simulink model "Motion_Planning"  (R2023b)
settings: Solver=VariableStepAuto  StartTime=0.0  StopTime=10.0  RelTol=1e-3
undefined symbols (not defined in the file or in its folder): Spline_Max_Centripital_Acceleration, Spline_Max_Linear_Acceleration, Spline_Max_Num_RefPoses, Spline_Max_Speed, Spline_Num_Samples
libraries: simulink x10
settings Model: Creator=FIRSTMentor  LastModifiedBy=FIRSTMentor

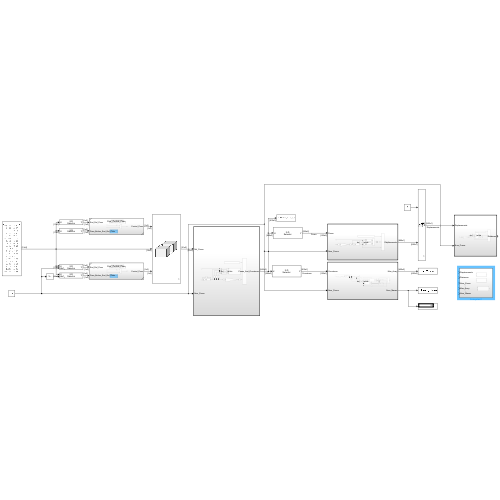
[thumbnail: Simulink's stored preview of the top-level diagram]
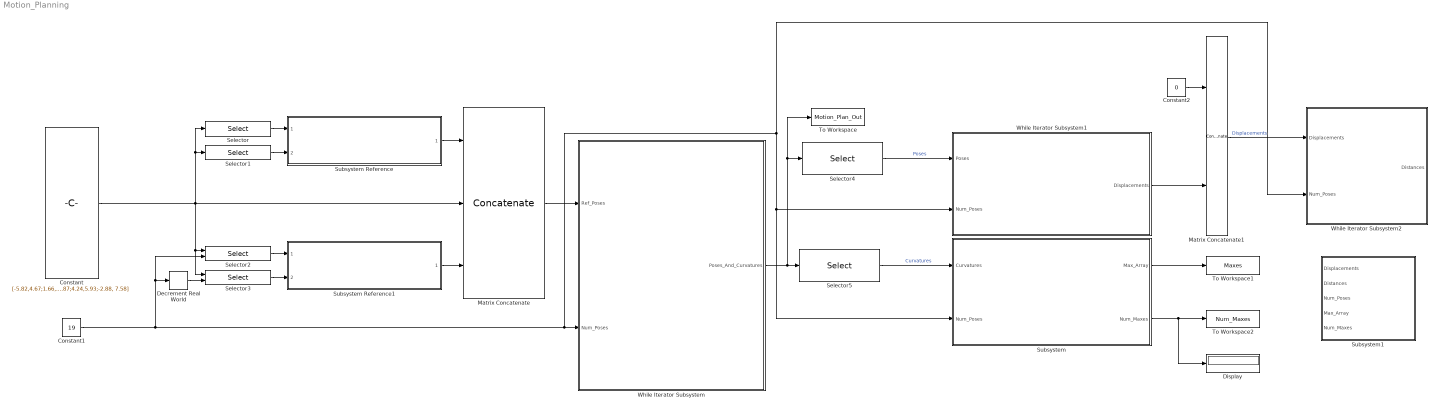
== system Motion_Planning ==
  Constant : Constant  Value=[-5.82,4.67;1.66,4.85;5,3.79;4.44,2.57;-5.94,2.47;-6.48,1.59;-5.46,0.81;4.2,0.75;-5.46,-0.25;3.9,-1.37;2.52,-2.81;5.36,-3.05;2.44,-4.71;-6.24,-4.09;-7.4,-2.43;-7.94,4.19;-7.6,5.87;4.24,5.93;-2.88, 7.58]  VectorParams1D=off
  Constant1 : Constant  Value=19
  Constant2 : Constant  Value=0
  Decrement Real World : simulink/Additional Math & Discrete/Additional Math: Increment - Decrement/Decrement Real World
  Display : Display
  Matrix Concatenate : Concatenate  NumInputs=3  Mode=Multidimensional array
  Matrix Concatenate1 : Concatenate  Mode=Multidimensional array
  Selector : Selector  NumberOfDimensions=2  InputPortWidth=3  IndexOptions=Index vector (dialog),Select all  Indices=1,1  OutputSizes=1,1
  Selector1 : Selector  NumberOfDimensions=2  InputPortWidth=3  IndexOptions=Index vector (dialog),Select all  Indices=2,1  OutputSizes=1,1
  Selector2 : Selector  NumberOfDimensions=2  InputPortWidth=3  IndexOptions=Index vector (port),Select all  Indices=[1 3],1  OutputSizes=1,1
  Selector3 : Selector  NumberOfDimensions=2  InputPortWidth=3  IndexOptions=Index vector (port),Select all  Indices=[1 3],1  OutputSizes=1,1
  Selector4 : Selector  NumberOfDimensions=2  InputPortWidth=3  IndexOptions=Select all,Index vector (dialog)  Indices=[1 3],[1,2]  OutputSizes=1,1
  Selector5 : Selector  NumberOfDimensions=2  InputPortWidth=3  IndexOptions=Select all,Index vector (dialog)  Indices=[1 3],3  OutputSizes=1,1
  Subsystem : Subsystem
  Subsystem Reference : Subsystem  ReferencedSubsystem=Find_Control_Pose
  Subsystem Reference1 : Subsystem  ReferencedSubsystem=Find_Control_Pose
  Subsystem1 : Subsystem
  To Workspace : ToWorkspace  VariableName=Motion_Plan_Out  SampleTime=20
  To Workspace1 : ToWorkspace  VariableName=Maxes  SampleTime=20
  To Workspace2 : ToWorkspace  VariableName=Num_Maxes  SampleTime=20
  While Iterator Subsystem : Subsystem  TreatAsAtomicUnit=on
  While Iterator Subsystem1 : Subsystem  TreatAsAtomicUnit=on
  While Iterator Subsystem2 : Subsystem  TreatAsAtomicUnit=on
  wires:
  Constant/1 -> Selector/1, Selector1/1, Selector3/1, Selector2/1, Matrix Concatenate/2
  Constant1/1 -> While Iterator Subsystem2/2(Num_Poses), Subsystem/2(Num_Poses), While Iterator Subsystem1/2(Num_Poses), While Iterator Subsystem/2(Num_Poses), Decrement Real World/1, Selector2/2
  While Iterator Subsystem/1(Poses_And_Curvatures) -> Selector4/1, To Workspace/1, Selector5/1
  Matrix Concatenate/1 -> While Iterator Subsystem/1(Ref_Poses)
  Subsystem Reference1/1 -> Matrix Concatenate/3
  Subsystem Reference/1 -> Matrix Concatenate/1
  Selector1/1 -> Subsystem Reference/2
  Selector/1 -> Subsystem Reference/1
  Selector2/1 -> Subsystem Reference1/1
  Selector3/1 -> Subsystem Reference1/2
  Decrement Real World/1 -> Selector3/2
  Selector4/1 -> While Iterator Subsystem1/1(Poses)  "Poses"
  While Iterator Subsystem1/1(Displacements) -> Matrix Concatenate1/2
  Constant2/1 -> Matrix Concatenate1/1
  Selector5/1 -> Subsystem/1(Curvatures)  "Curvatures"
  Matrix Concatenate1/1 -> While Iterator Subsystem2/1(Displacements)  "Displacements"
  Subsystem/1(Max_Array) -> To Workspace1/1
  Subsystem/2(Num_Maxes) -> To Workspace2/1, Display/1

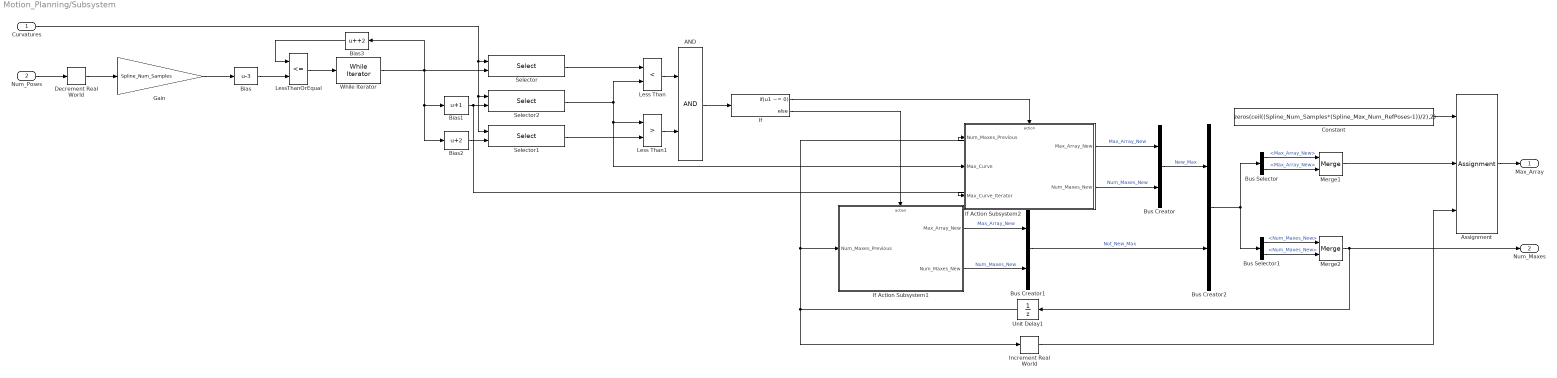
== system Motion_Planning/Subsystem ==
  Curvatures : Inport
  Num_Poses : Inport  Port=2
  AND : Logic  AllPortsSameDT=off  OutDataTypeStr=boolean
  Assignment : Assignment  NumberOfDimensions=2  DiagnosticForDimensions=Warning  IndexOptions=Index vector (port),Assign all  Indices=1,1  OutputSizes=1,1
  Bias : Bias  Bias=-3  SaturateOnIntegerOverflow=off
  Bias1 : Bias  Bias=1  SaturateOnIntegerOverflow=off
  Bias2 : Bias  Bias=2  SaturateOnIntegerOverflow=off
  Bias3 : Bias  Bias=+2  SaturateOnIntegerOverflow=off
  Bus Creator : BusCreator  Inputs=2
  Bus Creator1 : BusCreator  Inputs=2
  Bus Creator2 : BusCreator  Inputs=2
  Bus Selector : BusSelector  OutputSignals=New_Max.Max_Array_New,Not_New_Max.Max_Array_New
  Bus Selector1 : BusSelector  OutputSignals=New_Max.Num_Maxes_New,Not_New_Max.Num_Maxes_New
  Constant : Constant  Value=zeros(ceil((Spline_Num_Samples*(Spline_Max_Num_RefPoses-1))/2),2)
  Decrement Real World : simulink/Additional Math & Discrete/Additional Math: Increment - Decrement/Decrement Real World
  Gain : Gain  Gain=Spline_Num_Samples
  If : If  IfExpression=u1 ~= 0
  If Action Subsystem1 : Subsystem  TreatAsAtomicUnit=on
  If Action Subsystem2 : Subsystem  TreatAsAtomicUnit=on
  Increment Real World : simulink/Additional Math & Discrete/Additional Math: Increment - Decrement/Increment Real World
  Less Than : RelationalOperator  Operator=<  OutDataTypeStr=boolean  RndMeth=Simplest  InputSameDT=off
  Less Than1 : RelationalOperator  Operator=>  OutDataTypeStr=boolean  RndMeth=Simplest  InputSameDT=off
  LessThanOrEqual : RelationalOperator  Operator=<=  OutDataTypeStr=boolean  RndMeth=Simplest  InputSameDT=off
  Merge1 : Merge
  Merge2 : Merge
  Selector : Selector  NumberOfDimensions=2  InputPortWidth=3  IndexOptions=Index vector (port),Select all  Indices=[1 3],1  OutputSizes=1,1
  Selector1 : Selector  NumberOfDimensions=2  InputPortWidth=3  IndexOptions=Index vector (port),Select all  Indices=[1 3],1  OutputSizes=1,1
  Selector2 : Selector  NumberOfDimensions=2  InputPortWidth=3  IndexOptions=Index vector (port),Select all  Indices=[1 3],1  OutputSizes=1,1
  Unit Delay1 : UnitDelay  SampleTime=-1  HasFrameUpgradeWarning=on
  While Iterator : WhileIterator  MaxIters=Spline_Num_Samples*(Spline_Max_Num_RefPoses-1)-2  WhileBlockType=do-while  ShowIterationPort=on  OutputDataType=double
  Max_Array : Outport
  Num_Maxes : Outport  Port=2
  wires:
  LessThanOrEqual/1 -> While Iterator/1
  Num_Poses/1 -> Decrement Real World/1
  Decrement Real World/1 -> Gain/1
  Gain/1 -> Bias/1
  Bias/1 -> LessThanOrEqual/2
  While Iterator/1 -> Bias3/1, Bias1/1, Bias2/1, Selector/2
  Bias1/1 -> If Action Subsystem2/3(Max_Curve_Iterator), Selector2/2
  Bias2/1 -> Selector1/2
  Curvatures/1 -> Selector/1, Selector2/1, Selector1/1
  Bias3/1 -> LessThanOrEqual/1
  Selector2/1 -> If Action Subsystem2/2(Max_Curve), Less Than1/1, Less Than/2
  Selector/1 -> Less Than/1
  Selector1/1 -> Less Than1/2
  Less Than/1 -> AND/1
  Less Than1/1 -> AND/2
  AND/1 -> If/1
  If/1 -> If Action Subsystem2/Action
  If/2 -> If Action Subsystem1/Action
  If Action Subsystem2/2(Num_Maxes_New) -> Bus Creator/2  "Num_Maxes_New"
  If Action Subsystem2/1(Max_Array_New) -> Bus Creator/1  "Max_Array_New"
  If Action Subsystem1/1(Max_Array_New) -> Bus Creator1/1  "Max_Array_New"
  If Action Subsystem1/2(Num_Maxes_New) -> Bus Creator1/2  "Num_Maxes_New"
  Bus Creator1/1 -> Bus Creator2/2  "Not_New_Max"
  Bus Creator/1 -> Bus Creator2/1  "New_Max"
  Bus Selector/1 -> Merge1/1  "<Max_Array_New>"
  Bus Selector/2 -> Merge1/2  "<Max_Array_New>"
  Bus Selector1/2 -> Merge2/2  "<Num_Maxes_New>"
  Bus Selector1/1 -> Merge2/1  "<Num_Maxes_New>"
  Bus Creator2/1 -> Bus Selector/1, Bus Selector1/1
  Merge1/1 -> Assignment/2
  Merge2/1 -> Num_Maxes/1, Unit Delay1/1
  Unit Delay1/1 -> Increment Real World/1, If Action Subsystem2/1(Num_Maxes_Previous), If Action Subsystem1/1(Num_Maxes_Previous)
  Assignment/1 -> Max_Array/1
  Increment Real World/1 -> Assignment/3
  Constant/1 -> Assignment/1

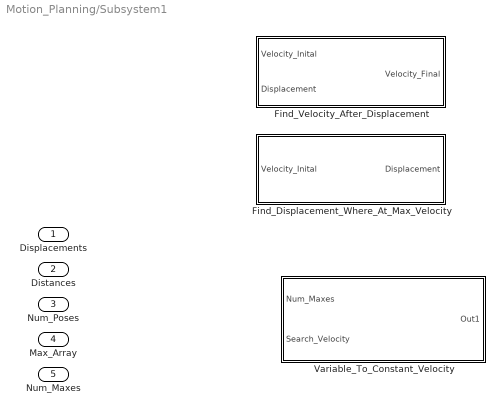
== system Motion_Planning/Subsystem1 ==
  Displacements : Inport
  Distances : Inport  Port=2
  Num_Poses : Inport  Port=3
  Max_Array : Inport  Port=4
  Num_Maxes : Inport  Port=5
  Find_Displacement_Where_At_Max_Velocity : Subsystem
  Find_Velocity_After_Displacement : Subsystem
  Variable_To_Constant_Velocity : Subsystem  TreatAsAtomicUnit=on

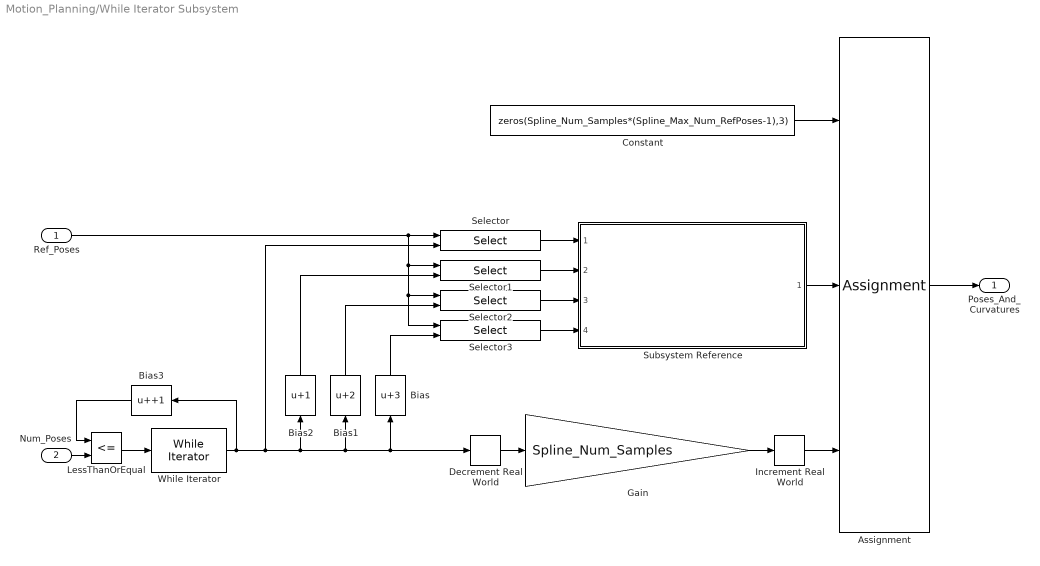
== system Motion_Planning/While Iterator Subsystem ==
  Ref_Poses : Inport
  Num_Poses : Inport  Port=2
  Assignment : Assignment  NumberOfDimensions=2  DiagnosticForDimensions=Warning  IndexOptions=Starting index (port),Assign all  Indices=1,1  OutputSizes=1,1
  Bias : Bias  Bias=3  SaturateOnIntegerOverflow=off
  Bias1 : Bias  Bias=2  SaturateOnIntegerOverflow=off
  Bias2 : Bias  Bias=1  SaturateOnIntegerOverflow=off
  Bias3 : Bias  Bias=+1  SaturateOnIntegerOverflow=off
  Constant : Constant  Value=zeros(Spline_Num_Samples*(Spline_Max_Num_RefPoses-1),3)  VectorParams1D=off
  Decrement Real World : simulink/Additional Math & Discrete/Additional Math: Increment - Decrement/Decrement Real World
  Gain : Gain  Gain=Spline_Num_Samples
  Increment Real World : simulink/Additional Math & Discrete/Additional Math: Increment - Decrement/Increment Real World
  LessThanOrEqual : RelationalOperator  Operator=<=  OutDataTypeStr=boolean  RndMeth=Simplest  InputSameDT=off
  Selector{,1..3} (4 alike) : Selector  NumberOfDimensions=2  InputPortWidth=3  IndexOptions=Index vector (port),Select all  Indices=[1 3],1  OutputSizes=1,1
  Subsystem Reference : Subsystem  ReferencedSubsystem=Sample_Catmull_Rom_Pos_And_Curve
  While Iterator : WhileIterator  MaxIters=Spline_Max_Num_RefPoses-1  WhileBlockType=do-while  ShowIterationPort=on  OutputDataType=double
  Poses_And_Curvatures : Outport
  wires:
  Selector/1 -> Subsystem Reference/1
  Selector1/1 -> Subsystem Reference/2
  Selector2/1 -> Subsystem Reference/3
  Selector3/1 -> Subsystem Reference/4
  Ref_Poses/1 -> Selector3/1, Selector2/1, Selector1/1, Selector/1
  While Iterator/1 -> Bias3/1, Selector/2, Bias2/1, Bias1/1, Decrement Real World/1, Bias/1
  Bias/1 -> Selector3/2
  Bias1/1 -> Selector2/2
  Bias2/1 -> Selector1/2
  LessThanOrEqual/1 -> While Iterator/1
  Num_Poses/1 -> LessThanOrEqual/2
  Subsystem Reference/1 -> Assignment/2
  Gain/1 -> Increment Real World/1
  Constant/1 -> Assignment/1
  Assignment/1 -> Poses_And_Curvatures/1
  Bias3/1 -> LessThanOrEqual/1
  Decrement Real World/1 -> Gain/1
  Increment Real World/1 -> Assignment/3

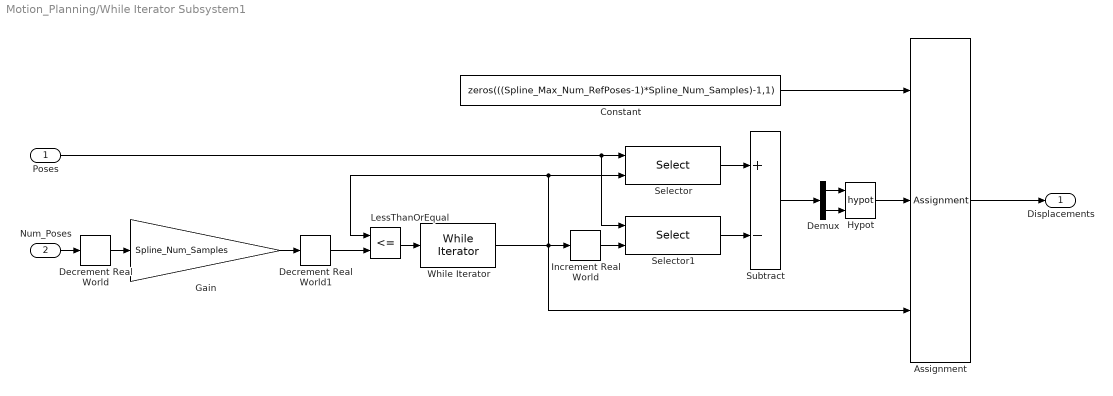
== system Motion_Planning/While Iterator Subsystem1 ==
  Poses : Inport
  Num_Poses : Inport  Port=2
  Assignment : Assignment  NumberOfDimensions=2  DiagnosticForDimensions=Warning  IndexOptions=Index vector (port),Assign all  Indices=1,1  OutputSizes=1,1
  Constant : Constant  Value=zeros(((Spline_Max_Num_RefPoses-1)*Spline_Num_Samples)-1,1)  VectorParams1D=off
  Decrement Real World : simulink/Additional Math & Discrete/Additional Math: Increment - Decrement/Decrement Real World
  Decrement Real World1 : simulink/Additional Math & Discrete/Additional Math: Increment - Decrement/Decrement Real World
  Demux : Demux  Outputs=2
  Gain : Gain  Gain=Spline_Num_Samples
  Hypot : Math  Operator=hypot
  Increment Real World : simulink/Additional Math & Discrete/Additional Math: Increment - Decrement/Increment Real World
  LessThanOrEqual : RelationalOperator  Operator=<=  OutDataTypeStr=boolean  RndMeth=Simplest  InputSameDT=off
  Selector : Selector  NumberOfDimensions=2  InputPortWidth=3  IndexOptions=Index vector (port),Select all  Indices=[1 3],1  OutputSizes=1,1
  Selector1 : Selector  NumberOfDimensions=2  InputPortWidth=3  IndexOptions=Index vector (port),Select all  Indices=[1 3],1  OutputSizes=1,1
  Subtract : Sum  Inputs=+-
  While Iterator : WhileIterator  WhileBlockType=do-while  ShowIterationPort=on
  Displacements : Outport
  wires:
  Poses/1 -> Selector1/1, Selector/1
  While Iterator/1 -> Assignment/3, Increment Real World/1, LessThanOrEqual/1, Selector/2
  Increment Real World/1 -> Selector1/2
  LessThanOrEqual/1 -> While Iterator/1
  Num_Poses/1 -> Decrement Real World/1
  Decrement Real World/1 -> Gain/1
  Gain/1 -> Decrement Real World1/1
  Decrement Real World1/1 -> LessThanOrEqual/2
  Selector/1 -> Subtract/1
  Selector1/1 -> Subtract/2
  Subtract/1 -> Demux/1
  Demux/1 -> Hypot/1
  Demux/2 -> Hypot/2
  Hypot/1 -> Assignment/2
  Constant/1 -> Assignment/1
  Assignment/1 -> Displacements/1

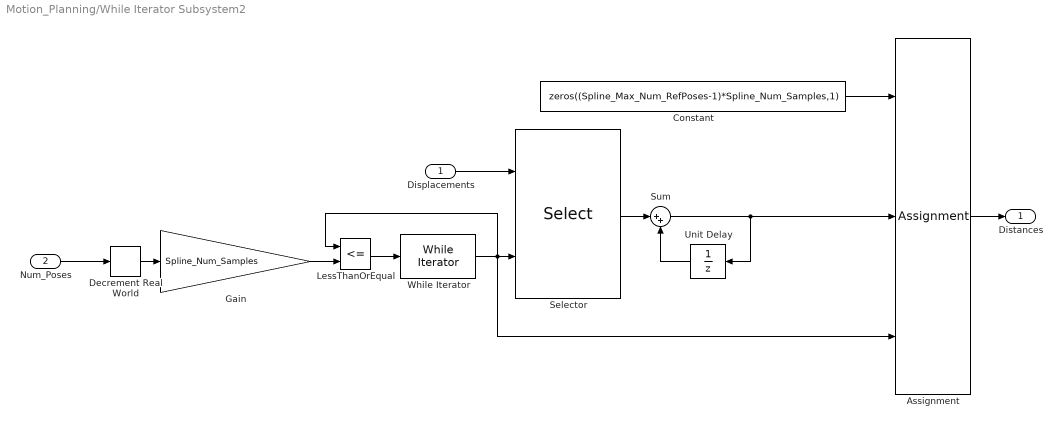
== system Motion_Planning/While Iterator Subsystem2 ==
  Displacements : Inport
  Num_Poses : Inport  Port=2
  Assignment : Assignment  NumberOfDimensions=2  DiagnosticForDimensions=Warning  IndexOptions=Index vector (port),Assign all  Indices=1,1  OutputSizes=1,1
  Constant : Constant  Value=zeros((Spline_Max_Num_RefPoses-1)*Spline_Num_Samples,1)
  Decrement Real World : simulink/Additional Math & Discrete/Additional Math: Increment - Decrement/Decrement Real World
  Gain : Gain  Gain=Spline_Num_Samples
  LessThanOrEqual : RelationalOperator  Operator=<=  OutDataTypeStr=boolean  RndMeth=Simplest  InputSameDT=off
  Selector : Selector  NumberOfDimensions=2  InputPortWidth=3  IndexOptions=Index vector (port),Select all  Indices=[1 3],1  OutputSizes=1,1
  Sum : Sum  Inputs=|++
  Unit Delay : UnitDelay  SampleTime=-1  HasFrameUpgradeWarning=on
  While Iterator : WhileIterator  WhileBlockType=do-while  ShowIterationPort=on  OutputDataType=double
  Distances : Outport
  wires:
  Assignment/1 -> Distances/1
  Displacements/1 -> Selector/1
  Selector/1 -> Sum/1
  Unit Delay/1 -> Sum/2
  Sum/1 -> Assignment/2, Unit Delay/1
  While Iterator/1 -> Assignment/3, LessThanOrEqual/1, Selector/2
  LessThanOrEqual/1 -> While Iterator/1
  Decrement Real World/1 -> Gain/1
  Gain/1 -> LessThanOrEqual/2
  Num_Poses/1 -> Decrement Real World/1
  Constant/1 -> Assignment/1

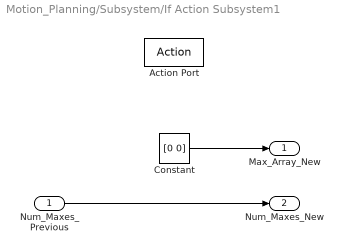
== system Motion_Planning/Subsystem/If Action Subsystem1 ==
  Num_Maxes_Previous : Inport
  Action Port : ActionPort  ActionPortLabel=else
  Constant : Constant  Value=[0 0]  VectorParams1D=off
  Max_Array_New : Outport
  Num_Maxes_New : Outport  Port=2
  wires:
  Num_Maxes_Previous/1 -> Num_Maxes_New/1
  Constant/1 -> Max_Array_New/1

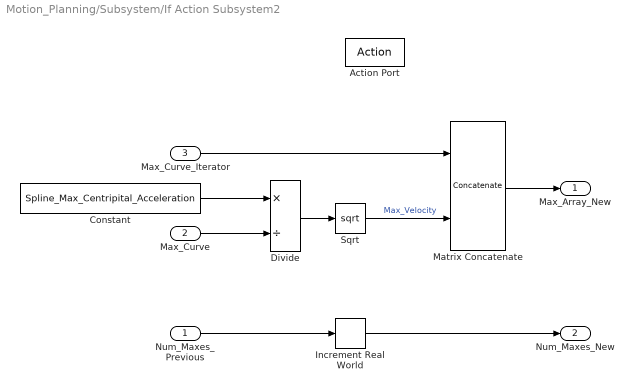
== system Motion_Planning/Subsystem/If Action Subsystem2 ==
  Num_Maxes_Previous : Inport
  Max_Curve : Inport  Port=2
  Max_Curve_Iterator : Inport  Port=3
  Action Port : ActionPort  ActionPortLabel=if(u1 ~= 0)
  Constant : Constant  Value=Spline_Max_Centripital_Acceleration
  Divide : Product  Inputs=*/
  Increment Real World : simulink/Additional Math & Discrete/Additional Math: Increment - Decrement/Increment Real World
  Matrix Concatenate : Concatenate  Mode=Multidimensional array  ConcatenateDimension=2
  Sqrt : Sqrt
  Max_Array_New : Outport
  Num_Maxes_New : Outport  Port=2
  wires:
  Num_Maxes_Previous/1 -> Increment Real World/1
  Increment Real World/1 -> Num_Maxes_New/1
  Matrix Concatenate/1 -> Max_Array_New/1
  Divide/1 -> Sqrt/1
  Sqrt/1 -> Matrix Concatenate/2  "Max_Velocity"
  Constant/1 -> Divide/1
  Max_Curve_Iterator/1 -> Matrix Concatenate/1
  Max_Curve/1 -> Divide/2

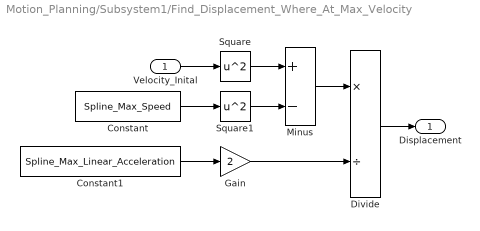
== system Motion_Planning/Subsystem1/Find_Displacement_Where_At_Max_Velocity ==
  Velocity_Inital : Inport
  Constant : Constant  Value=Spline_Max_Speed
  Constant1 : Constant  Value=Spline_Max_Linear_Acceleration
  Divide : Product  Inputs=*/
  Gain : Gain  Gain=2
  Minus : Sum  Inputs=+-
  Square : Math  Operator=square
  Square1 : Math  Operator=square
  Displacement : Outport
  wires:
  Velocity_Inital/1 -> Square/1
  Constant/1 -> Square1/1
  Square/1 -> Minus/1
  Square1/1 -> Minus/2
  Constant1/1 -> Gain/1
  Gain/1 -> Divide/2
  Minus/1 -> Divide/1
  Divide/1 -> Displacement/1

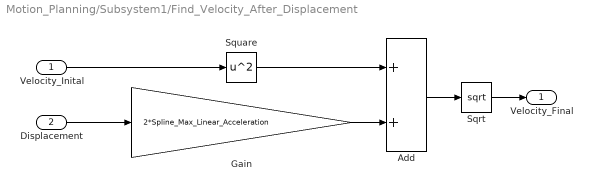
== system Motion_Planning/Subsystem1/Find_Velocity_After_Displacement ==
  Velocity_Inital : Inport
  Displacement : Inport  Port=2
  Add : Sum
  Gain : Gain  Gain=2*Spline_Max_Linear_Acceleration
  Sqrt : Sqrt
  Square : Math  Operator=square
  Velocity_Final : Outport
  wires:
  Velocity_Inital/1 -> Square/1
  Displacement/1 -> Gain/1
  Square/1 -> Add/1
  Gain/1 -> Add/2
  Add/1 -> Sqrt/1
  Sqrt/1 -> Velocity_Final/1

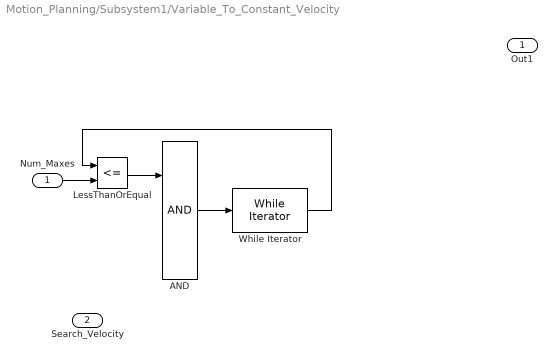
== system Motion_Planning/Subsystem1/Variable_To_Constant_Velocity ==
  Num_Maxes : Inport
  Search_Velocity : Inport  Port=2
  AND : Logic  AllPortsSameDT=off  OutDataTypeStr=boolean
  LessThanOrEqual : RelationalOperator  Operator=<=  OutDataTypeStr=boolean  RndMeth=Simplest  InputSameDT=off
  While Iterator : WhileIterator  WhileBlockType=do-while  ShowIterationPort=on  OutputDataType=double
  Out1 : Outport
  wires:
  While Iterator/1 -> LessThanOrEqual/1
  Num_Maxes/1 -> LessThanOrEqual/2
  LessThanOrEqual/1 -> AND/1
  AND/1 -> While Iterator/1
